simulink model "model_1"  (R2016b)
settings: Solver=VariableStepAuto  StartTime=0.0  StopTime=2  RelTol=1e-3
undefined symbols (not defined in the file): DiscIntNeverNeededParam
libraries: powerlib x10, simulink_need_slupdate x2, simulink x1
settings Model: Creator=sithuaung  LastModifiedBy=sithuaung

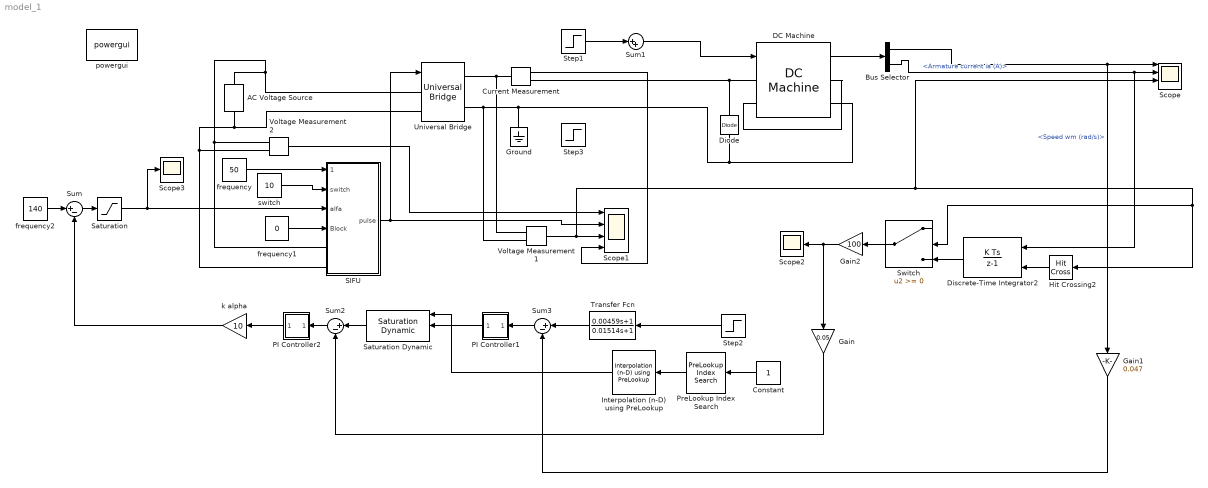
== system model_1 ==
  AC Voltage Source : powerlib/Electrical Sources/AC Voltage Source  Amplitude=220*sqrt(2)  Phase=0  Frequency=50  SampleTime=0  Measurements=None  BusType=swing  Pref=10e3  Qref=0  Qmin=-inf  Qmax=+inf
  Bus Selector : BusSelector  OutputSignals=Speed wm (rad/s),Armature current ia (A)
  Constant : Constant
  Current Measurement : powerlib/Measurements/Current Measurement  PhasorSimulation=off  OutputType=Complex  PSBequivalent=0
  DC Machine : powerlib/Machines/DC Machine  PresetModel=No  MechanicalLoad=Torque TL  FieldType=Wound  ShowDetailedParameters=on  MeasurementBus=off  RLa="[ 7.061  0.058]"  RLf="[ 12.939  0.531]"  Laf=0.0662  MachineConstant=Torque constant (N.m/A)  Ke=1.8  Kt=1.8  J=0.21e-3  Bm=0  Tf=0  w0=1  Ifinit=-8.46539071434242e-022  TsPowergui=0  TsBlock=-1
      settings: AttributesFormatString=\n
  Diode : powerlib/Power Electronics/Diode  Ron=0.001  Lon=0  Vf=0.8  IC=0  UseSnubber=off  Rs=inf  Cs=inf  Measurements=off
  Discrete-Time Integrator2 : DiscreteIntegrator  gainval=1  ExternalReset=rising  SampleTime=2e-005  ICPrevOutput=DiscIntNeverNeededParam  ICPrevScaledInput=DiscIntNeverNeededParam
  Gain : Gain  Gain=0.05
  Gain1 : Gain  Gain=0.047
  Gain2 : Gain  Gain=100
  Ground : powerlib/Elements/Ground  LConnTagsString=a
  Hit Crossing2 : HitCross  HitCrossingDirection=rising  SampleTime=2e-005
  Interpolation (n-D) using PreLookup : simulink_need_slupdate/Interpolation (n-D) using PreLookup  numDimsPopupSelect=1  explicitNumDims=2  table=[10 10 9.2 4.72 3.02 2.075 2.075]  interpMethod=Linear  extrapMethod=Linear  rangeErrorMode=None  NumSelectionDims=0
  PI Controller1 : Subsystem  AncestorBlock=simulink_extras/Additional Linear/PID Controller  mask(PI Controller){P=10, I=1/0.01514}
      mask prompts: P "Proportional:"; I "Integral I:"
      mask help:
      | Enter expressions for proportional and integral  terms.
      | P*(1+I/s)
      mask Help: This block implements a PID controller where parameters are entered for the Proportional, Integral and Derivative terms. Unmask this block to see how it works. The derivative term is implemented using a true derivative block.
      mask Display: disp('PI')
  PI Controller2 : Subsystem  AncestorBlock=simulink_extras/Additional Linear/PID Controller  mask(PI Controller){P=1, I=180}
      mask prompts: P "Proportional:"; I "Integral I:"
      mask help:
      | Enter expressions for proportional and integral  terms.
      | P*(1+I/s)
      mask Help: This block implements a PID controller where parameters are entered for the Proportional, Integral and Derivative terms. Unmask this block to see how it works. The derivative term is implemented using a true derivative block.
      mask Display: disp('PI')
  PreLookup Index Search : simulink_need_slupdate/PreLookup Index Search  bpData=[0 27.3 52.5 105 157.5 210 262.5]  searchMode=Binary Search  cacheBpFlag=off  outputFlag=off  IndexDataType=uint32  extrapMode=Linear Extrapolation  rangeErrorMode=None
  SIFU : Subsystem
  Saturation : Saturate  UpperLimit=80  LowerLimit=20
  Saturation Dynamic : simulink/Discontinuities/Saturation Dynamic  OutMin=[]  OutMax=[]  OutDataTypeStr=Inherit: Same as second input  OutDataType=fixdt(1, 16)  OutScaling=2^-10  DoSatur=off
  Scope : Scope  NumInputPorts=4
  Scope1 : Scope  NumInputPorts=4
  Scope2 : Scope
  Scope3 : Scope
  Step1 : Step  Time=0  After=0.226  SampleTime=0
  Step2 : Step  Time=0  After=30  SampleTime=0
  Step3 : Step  After=0.5  SampleTime=0
  Sum : Sum  Inputs=|+-
  Sum1 : Sum  Inputs=|++
  Sum2 : Sum  Inputs=|+-
  Sum3 : Sum  Inputs=|+-
  Switch : Switch  ZeroCross=off
  Transfer Fcn : TransferFcn  Numerator=[0.00459 1]  Denominator=[0.01514 1]
  Universal Bridge : powerlib/Power Electronics/Universal Bridge  Arms=2  SnubberResistance=100  SnubberCapacitance=0.1e-6  Device=Thyristors  Ron=1e-3  Lon=0  ForwardVoltages="[  0  0  ]"  ForwardVoltage=0  GTOparameters=[ 10e-6 , 20e-6 ]  IGBTparameters=[ 1e-6 , 2e-6 ]  Measurements=None  Measurements_2=None  converterType=Rectifier
  Voltage Measurement1 : powerlib/Measurements/Voltage Measurement  PhasorSimulation=off  OutputType=Complex  PSBequivalent=0
  Voltage Measurement2 : powerlib/Measurements/Voltage Measurement  PhasorSimulation=off  OutputType=Complex  PSBequivalent=0
  frequency : Constant  Value=50
  frequency1 : Constant  Value=0
  frequency2 : Constant  Value=140
  k alpha : Gain  Gain=10  SaturateOnIntegerOverflow=on  OutDataTypeStr=Inherit: Same as input  ParamDataTypeStr=Inherit: Same as input
  powergui : powerlib/powergui  Priority=1  SimulationMode=Continuous  SolverType=Tustin/Backward Euler (TBE)  SampleTime=50e-6  frequency=60  SPID=off  DisableSnubberDevices=off  DisableRonSwitches=off  DisableVfSwitches=off  SwTol=0  DisplayEquations=off  Interpol=off  ExternalGateDelay=off  methode=off  Ts=10  FunctionMessages=off  echomessages=off  HookPort=off  EnableUseOfTLC=off  x0status=blocks  frequencyindice=50  Pbase=100e6  ErrMax=1e-4  Iterations=50  UnitsV=kV  UnitsW=MW  buscounter=0  RestoreLinks=warning  ResistiveCurrentMeasurement=off  Frange=[0:2:500]  Ylog=off  Xlog=on  ShowGrid=off  save=off  variable=ZData  structure=0  ZoomFFT=off  StartTime=0.0  cycles=1  DisplayStyle=1  fundamental=60  FreqAxis=off  MaxFrequency=1000  frequencyindicesteady=1  RmsSteady=1  display=off
  switch : Constant  Value=10
  wires:
  frequency/1 -> SIFU/1(frequency)
  switch/1 -> SIFU/2(switch)
  frequency1/1 -> SIFU/4(Block)
  Current Measurement/1 -> Scope1/4
  Voltage Measurement2/1 -> Scope1/1
  DC Machine/1 -> Bus Selector/1
  Bus Selector/1 -> Gain1/1, Scope/1  "<Speed wm (rad/s)>"
  Bus Selector/2 -> Discrete-Time Integrator2/1, Scope/2  "<Armature current ia (A)>"
  Sum3/1 -> PI Controller1/1(In_1)
  Sum2/1 -> PI Controller2/1(In_1)
  Transfer Fcn/1 -> Sum3/1
  PreLookup Index Search/1 -> Interpolation (n-D) using PreLookup/1
  PI Controller1/1(Out_1) -> Saturation Dynamic/2
  Saturation Dynamic/1 -> Sum2/1
  Gain/1 -> Sum2/2
  Gain1/1 -> Sum3/2
  PI Controller2/1(Out_1) -> k alpha/1
  frequency2/1 -> Sum/1
  Sum/1 -> Saturation/1
  k alpha/1 -> Sum/2
  Step2/1 -> Transfer Fcn/1
  Step1/1 -> Sum1/1
  Sum1/1 -> DC Machine/1
  Hit Crossing2/1 -> Discrete-Time Integrator2/2
  Discrete-Time Integrator2/1 -> Switch/3
  Switch/1 -> Gain2/1
  Gain2/1 -> Gain/1, Scope2/1
  SIFU/1(pulse) -> Universal Bridge/1, Scope1/2
  Voltage Measurement1/1 -> Scope/3, Hit Crossing2/1, Switch/2, Scope1/3
  Interpolation (n-D) using PreLookup/1 -> Saturation Dynamic/1
  Constant/1 -> PreLookup Index Search/1
  Saturation/1 -> Scope3/1, SIFU/3(alfa)
  connections:
  Universal Bridge/RConn1 -- Voltage Measurement1/LConn1 -- Current Measurement/LConn1
  Diode/LConn1 -- DC Machine/RConn2 -- Ground/LConn1 -- Voltage Measurement1/LConn2 -- Universal Bridge/RConn2
  Voltage Measurement2/LConn2 -- Universal Bridge/LConn2 -- AC Voltage Source/LConn1 -- SIFU/LConn2
  Voltage Measurement2/LConn1 -- Universal Bridge/LConn1 -- AC Voltage Source/RConn1 -- SIFU/LConn1
  DC Machine/LConn1 -- Diode/RConn1 -- Current Measurement/RConn1
  DC Machine/RConn1 -- DC Machine/LConn2

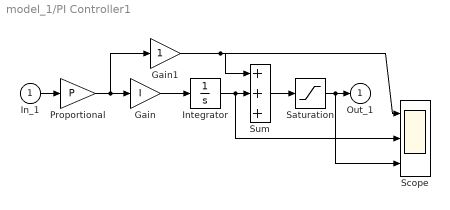
== system model_1/PI Controller1 ==
  In_1 : Inport
  Gain : Gain  Gain=I
  Gain1 : Gain
  Integrator : Integrator  LimitOutput=on  UpperSaturationLimit=3.16  LowerSaturationLimit=-3.16
  Proportional : Gain  Gain=P  SaturateOnIntegerOverflow=on  OutDataTypeStr=Inherit: Same as input  ParamDataTypeStr=Inherit: Same as input
  Saturation : Saturate  UpperLimit=10  LowerLimit=0
  Scope : Scope  NumInputPorts=3
  Sum : Sum  Inputs=+++  SaturateOnIntegerOverflow=on  InputSameDT=on  OutDataTypeStr=Inherit: Same as first input
  Out_1 : Outport  InitialOutput=0
  wires:
  Sum/1 -> Saturation/1
  In_1/1 -> Proportional/1
  Gain/1 -> Integrator/1
  Integrator/1 -> Sum/2, Scope/2
  Proportional/1 -> Gain/1, Gain1/1
  Gain1/1 -> Sum/1, Scope/1
  Saturation/1 -> Out_1/1, Scope/3

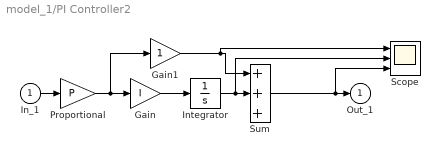
== system model_1/PI Controller2 ==
  In_1 : Inport
  Gain : Gain  Gain=I
  Gain1 : Gain
  Integrator : Integrator  LimitOutput=on  UpperSaturationLimit=6  LowerSaturationLimit=-6
  Proportional : Gain  Gain=P  SaturateOnIntegerOverflow=on  OutDataTypeStr=Inherit: Same as input  ParamDataTypeStr=Inherit: Same as input
  Scope : Scope  NumInputPorts=3
  Sum : Sum  Inputs=+++  SaturateOnIntegerOverflow=on  InputSameDT=on  OutDataTypeStr=Inherit: Same as first input
  Out_1 : Outport  InitialOutput=0
  wires:
  Sum/1 -> Out_1/1, Scope/3
  In_1/1 -> Proportional/1
  Gain/1 -> Integrator/1
  Integrator/1 -> Sum/2, Scope/2
  Proportional/1 -> Gain/1, Gain1/1
  Gain1/1 -> Sum/1, Scope/1

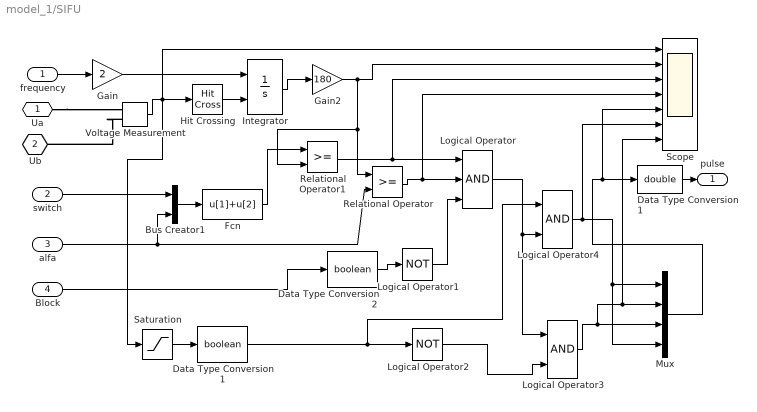
== system model_1/SIFU ==
  frequency : Inport
  switch : Inport  Port=2
  alfa : Inport  Port=3
  Block : Inport  Port=4
  Bus Creator1 : BusCreator  Inputs=2
  Data Type Conversion1 : DataTypeConversion  OutDataTypeStr=boolean  SaturateOnIntegerOverflow=on  RndMeth=Zero
  Data Type Conversion2 : DataTypeConversion  OutDataTypeStr=boolean  SaturateOnIntegerOverflow=on  RndMeth=Zero
  Data Type Conversion1 : DataTypeConversion  OutDataTypeStr=double
  Fcn : Fcn  Expr=u[1]+u[2]
  Gain : Gain  Gain=2
  Gain2 : Gain  Gain=180
  Hit Crossing : HitCross
  Integrator : Integrator  ExternalReset=either
  Logical Operator : Logic  Inputs=3  AllPortsSameDT=off  OutDataTypeStr=boolean
  Logical Operator1 : Logic  Operator=NOT  Inputs=3  AllPortsSameDT=off  OutDataTypeStr=boolean
  Logical Operator2 : Logic  Operator=NOT  Inputs=3  AllPortsSameDT=off  OutDataTypeStr=boolean
  Logical Operator3 : Logic  AllPortsSameDT=off  OutDataTypeStr=boolean
  Logical Operator4 : Logic  AllPortsSameDT=off  OutDataTypeStr=boolean
  Mux : Mux
  Relational Operator : RelationalOperator  OutDataTypeStr=boolean  RndMeth=Nearest
  Relational Operator1 : RelationalOperator  OutDataTypeStr=boolean  RndMeth=Nearest
  Saturation : Saturate  UpperLimit=1  LowerLimit=0
  Scope : Scope  NumInputPorts=7
  Voltage Measurement : powerlib/Measurements/Voltage Measurement  PhasorSimulation=off  OutputType=Complex  PSBequivalent=0
  Ua : PMIOPort  Port=1  Side=Left
  Ub : PMIOPort  Port=2  Side=Left
  pulse : Outport
  wires:
  Integrator/1 -> Gain2/1
  Hit Crossing/1 -> Integrator/2
  Gain2/1 -> Scope/2, Relational Operator/1, Relational Operator1/2
  alfa/1 -> Bus Creator1/2, Relational Operator/2
  Bus Creator1/1 -> Fcn/1
  Fcn/1 -> Relational Operator1/1
  Relational Operator1/1 -> Logical Operator/1, Scope/3
  Relational Operator/1 -> Logical Operator/2, Scope/4
  Voltage Measurement/1 -> Hit Crossing/1, Scope/1, Saturation/1
  frequency/1 -> Gain/1
  Data Type Conversion1/1 -> pulse/1
  switch/1 -> Bus Creator1/1
  Gain/1 -> Integrator/1
  Block/1 -> Data Type Conversion2/1
  Data Type Conversion2/1 -> Logical Operator1/1
  Logical Operator1/1 -> Logical Operator/3
  Saturation/1 -> Data Type Conversion1/1
  Data Type Conversion1/1 -> Logical Operator2/1, Logical Operator4/1
  Logical Operator/1 -> Logical Operator4/2, Logical Operator3/1
  Logical Operator4/1 -> Mux/1, Mux/4, Scope/6
  Logical Operator3/1 -> Mux/3, Mux/2, Scope/7
  Mux/1 -> Data Type Conversion1/1, Scope/5
  Logical Operator2/1 -> Logical Operator3/2
  connections:
  Voltage Measurement/LConn2 -- Ub/RConn1
  Ua/RConn1 -- Voltage Measurement/LConn1
